simulink model "gm_uz_typeconv_27En18_to27En15"  (R2021a)
settings: Solver=FixedStepDiscrete  StartTime=0.0  StopTime=0.1  RelTol=1e-3
undefined symbols (not defined in the file or in its folder): t_ADC
libraries: simulink x1
settings Model: Creator=micha  LastModifiedBy=micha
settings SolverCC: AlgebraicLoopSolver=TrustRegion
settings DataIOCC: LimitDataPoints=on  SaveOutput=off  SaveTime=off
settings OptimizationCC: BlockReduction=off  ConditionallyExecuteInputs=off  DefaultParameterBehavior=Inlined  LifeSpan=inf
settings DebuggingCC: AlgebraicLoopMsg=error  InheritedTsInSrcMsg=none  SingleTaskRateTransMsg=error  AllowSymbolicDim=off  StrictBusMsg=ErrorOnBusTreatedAsVector  SFUnexpectedBacktrackingDiag=warning  SFNoUnconditionalDefaultTransitionDiag=warning  SFExecutionAtInitializationDiag=none  SFMachineParentedDataDiag=warning  ArithmeticOperatorsInVariantConditions=warning
settings HardwareCC: ProdBitPerPointer=32  ProdBitPerSizeT=32  ProdBitPerPtrDiffT=32  ProdLargestAtomicFloat=None  ProdIntDivRoundTo=Undefined  ProdEndianess=Unspecified  ProdWordSize=32  ProdHWDeviceType=ASIC/FPGA->ASIC/FPGA  ProdEqTarget=off
settings SFSimCC: SimUseLocalCustomCode=off  CustomCodeUndefinedFunction=UseInterfaceOnly
settings RTWCC: RTWUseLocalCustomCode=off
settings CodeAppCC: StateflowObjectComments=on
settings GRTTargetCC: TargetLangStandard=C89/C90 (ANSI)
settings ConfigComp: CovScope=ReferencedModels  CovMetricSettings=dw  CovSaveCumulativeToWorkspaceVar=on  CovSaveSingleToWorkspaceVar=on  CovExternalEMLEnable=off  CovSFcnEnable=off

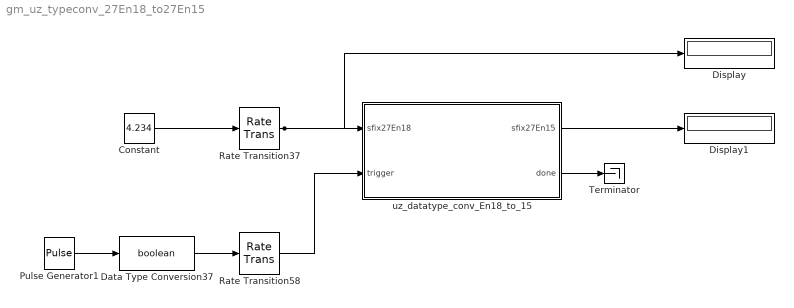
== system gm_uz_typeconv_27En18_to27En15 ==
  Constant : Constant  Value=4.234  OutDataTypeStr=fixdt(1,27,18)  SampleTime=-1
  Data Type Conversion37 : DataTypeConversion  OutDataTypeStr=boolean
  Display : Display
  Display1 : Display
  Pulse Generator1 : DiscretePulseGenerator  PulseType=Time based  Period=t_ADC  PulseWidth=5
  Rate Transition37 : RateTransition  OutPortSampleTime=t_clock
  Rate Transition58 : RateTransition  OutPortSampleTime=t_clock
  Terminator : Terminator
  uz_datatype_conv_En18_to_15 : Subsystem  TreatAsAtomicUnit=on
  wires:
  uz_datatype_conv_En18_to_15/2(done) -> Terminator/1
  Rate Transition37/1 -> uz_datatype_conv_En18_to_15/1(sfix27En18), Display/1
  Rate Transition58/1 -> uz_datatype_conv_En18_to_15/2(trigger)
  Pulse Generator1/1 -> Data Type Conversion37/1
  Data Type Conversion37/1 -> Rate Transition58/1
  uz_datatype_conv_En18_to_15/1(sfix27En15) -> Display1/1
  Constant/1 -> Rate Transition37/1

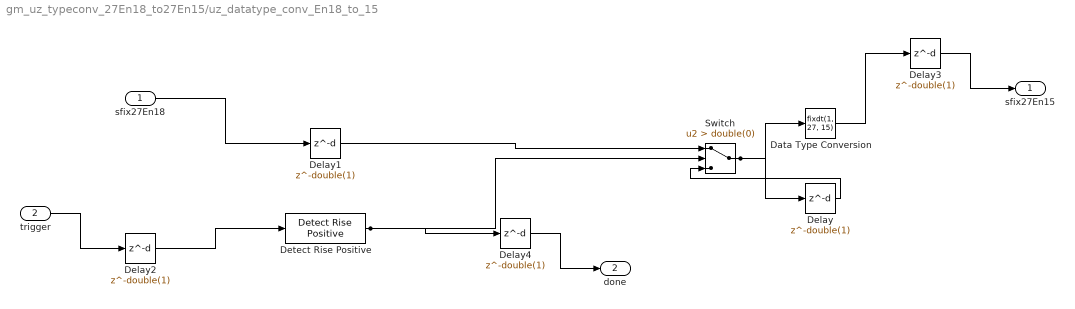
== system gm_uz_typeconv_27En18_to27En15/uz_datatype_conv_En18_to_15 ==
  sfix27En18 : Inport  OutDataTypeStr=fixdt(1, 27, 18)  PortDimensions=1  SampleTime=1e-08
  trigger : Inport  Port=2  OutDataTypeStr=boolean  PortDimensions=1  SampleTime=1e-08
  Data Type Conversion : DataTypeConversion  OutDataTypeStr=fixdt(1, 27, 15)  SampleTime=1e-08
  Delay{,1..4} (5 alike) : Delay  DelayLength=double(1)  InitialCondition=0  SampleTime=1e-08
  Detect Rise Positive : simulink/Logic and Bit Operations/Detect Rise Positive  vinit=0  OutDataTypeStr=boolean
  Switch : Switch  Criteria=u2 > Threshold  Threshold=double(0)  OutDataTypeStr=fixdt(1, 27, 18)  SampleTime=1e-08
  sfix27En15 : Outport  SampleTime=1e-08  VectorParamsAs1DForOutWhenUnconnected=off
  done : Outport  Port=2  SampleTime=1e-08  VectorParamsAs1DForOutWhenUnconnected=off
  wires:
  sfix27En18/1 -> Delay1/1
  trigger/1 -> Delay2/1
  Data Type Conversion/1 -> Delay3/1
  Delay/1 -> Switch/3
  Delay1/1 -> Switch/1
  Delay2/1 -> Detect Rise Positive/1
  Delay3/1 -> sfix27En15/1
  Delay4/1 -> done/1
  Detect Rise Positive/1 -> Switch/2, Delay4/1
  Switch/1 -> Data Type Conversion/1, Delay/1
